simulink model "slexHARiOSExample"  (R2021a)
settings: Solver=FixedStepDiscrete  StartTime=0.0  StopTime=Inf  RelTol=1e-3
model workspace (MAT data in the model file):
  jumpingImg = [255 255 255 255 255 255 255 255 255 255 255 255 ... (960000 elements, 800x400x3)]
  runningImg = [255 255 255 255 255 255 255 255 255 255 255 255 ... (960000 elements, 800x400x3)]
  sittingImg = [255 255 255 255 255 255 255 255 255 255 255 255 ... (960000 elements, 800x400x3)]
  standingImg = [255 255 255 255 255 255 255 255 255 255 255 255 ... (960000 elements, 800x400x3)]
  walkingImg = [255 255 255 255 255 255 255 255 255 255 255 255 ... (960000 elements, 800x400x3)]
values from neighbouring files (symbols this model uses):
  X = meas(:,1:2)    [ClusteringUsingGaussianMixtureModelsExample.m]    (also in ComputePairwiseDistance2UsingACustomDistanceFunctionExample.m = rand(3,3); EstimatePosteriorClassProbabilitiesECOCExample.m = X'; FittingGaussianProcessRegressionModelsToLargeDatasetsExample.m = [X,X.^2]; ModelswithCorrelatedandUncorrelatedRandomEffectsExample.m = [ones(406,1) Acceleration Horsepower])
  Y = tsne(X,'Algorithm','barneshut','NumPCAComponents',50)    [ChangeTsneSettingsExample.m]    (also in ComputePairwiseDistance2UsingACustomDistanceFunctionExample.m = [X(:,1:2) rand(3,1)]; TSNEOutputFunctionExample.m = tsne(meas,'Options',opts,'Algorithm','exact'); TuneGaussianMixtureModelsExample.m = zeros(n,1); VisualizeHighDimensionalDataUsingTSNEExample.m)
  Z = {ones(406,1),Acceleration}    [ModelswithCorrelatedandUncorrelatedRandomEffectsExample.m]
undefined symbols (not defined in the file or in its folder): Data_Display, HAR_app_ios
libraries: iosuilib x4, iosaudiovideolib x1, iossensorlib x1
(part 1 of 2)
settings Model: Creator=The MathWorks, Inc.  LastModifiedBy=The MathWorks, Inc.
settings SolverCC: AlgebraicLoopSolver=TrustRegion  MinimalZcImpactIntegration=on
settings DataIOCC: ReturnWorkspaceOutputs=off
settings OptimizationCC: PassReuseOutputArgsAs=Individual arguments  MaxStackSize=64  EfficientTunableParamExpr=on
settings DebuggingCC: ParameterTunabilityLossMsg=error  SFMachineParentedDataDiag=warning  ArithmeticOperatorsInVariantConditions=warning
settings HardwareCC: ProdBitPerPointer=32  ProdBitPerSizeT=32  ProdBitPerPtrDiffT=32  ProdLargestAtomicInteger=Long  ProdLargestAtomicFloat=Double  ProdWordSize=32  ProdHWDeviceType=ARM Compatible->ARM Cortex
settings SFSimCC: SimUseLocalCustomCode=off  MATLABDynamicMemAlloc=off
settings RTWCC: SystemTargetFile=ert.tlc  HardwareBoard=Apple iOS Device  TLCOptions="-aInlineSetEventsForThisBaseRateFcn=TLC_FALSE -aSuppressMultiTaskScheduler=TLC_FALSE  -aRateBasedStepFcn=0"  TemplateMakefile=ert_default_tmf  GenerateReport=on  RTWUseLocalCustomCode=off  Toolchain=Xcode iOS Project  BuildConfiguration=Faster Runs  LaunchReport=on
settings CodeAppCC: ForceParamTrailComments=on  IgnoreCustomStorageClasses=off  OperatorAnnotations=on  SimulinkDataObjDesc=on  SFDataObjDesc=on  MATLABFcnDesc=on  InsertBlockDesc=on  StateflowObjectComments=on  MATLABSourceComments=on
settings ERTTargetCC: SupportVariableSizeSignals=on  RootIOFormat=Structure reference

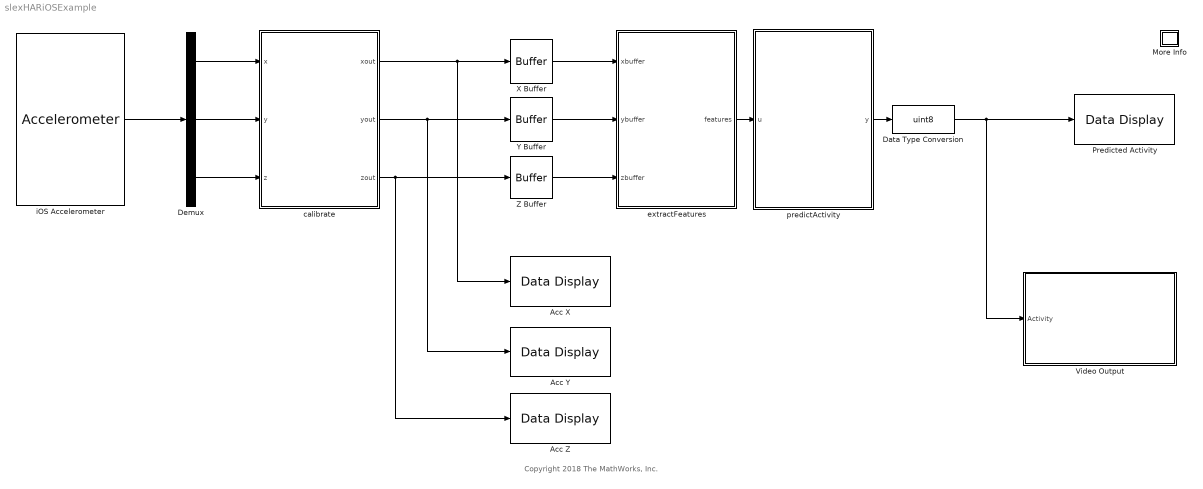
== system slexHARiOSExample ==
  note: Copyright 2018 The MathWorks, Inc.
  Acc X : iosuilib/Data Display  DataDisplayId=HAR_app_ios/X  Format=Float  Precision=6  SimulateUsing=Code generation  BlockPlatform=iOS
      settings: SourceProductBaseCode=SL_IOS
  Acc Y : iosuilib/Data Display  DataDisplayId=HAR_app_ios/Y  Format=Float  Precision=6  SimulateUsing=Code generation  BlockPlatform=iOS
      settings: SourceProductBaseCode=SL_IOS
  Acc Z : iosuilib/Data Display  DataDisplayId=HAR_app_ios/Z  Format=Float  Precision=6  SimulateUsing=Code generation  BlockPlatform=iOS
      settings: SourceProductBaseCode=SL_IOS
  Data Type Conversion : DataTypeConversion  OutDataTypeStr=uint8
  Demux : Demux  Outputs=3
  More Info : Subsystem
      settings: OpenFcn=showExample('stats/HARDeploymentExample')
      mask Display: disp('?')
  Predicted Activity : iosuilib/Data Display  DataDisplayId=HAR_app_ios/Data_Display  Format=Float  Precision=6  SimulateUsing=Code generation  BlockPlatform=iOS
      settings: SourceProductBaseCode=SL_IOS
  Video Output : Subsystem
  X Buffer : Buffer  N=32  V=12  OutputFrames=off
  Y Buffer : Buffer  N=32  V=12  OutputFrames=off
  Z Buffer : Buffer  N=32  V=12  OutputFrames=off
  calibrate : MATLAB Function  TreatAsAtomicUnit=on
  extractFeatures : MATLAB Function  TreatAsAtomicUnit=on
  iOS Accelerometer : iossensorlib/Accelerometer  OutputVector_=on  SampleTime_=0.1  blockPlatform=iOS
      settings: SourceProductBaseCode=SL_IOS
  predictActivity : MATLAB Function  TreatAsAtomicUnit=on
  wires:
  Data Type Conversion/1 -> Predicted Activity/1, Video Output/1(Activity)
  calibrate/3(zout) -> Acc Z/1, Z Buffer/1
  Y Buffer/1 -> extractFeatures/2(ybuffer)
  extractFeatures/1(features) -> predictActivity/1(u)
  X Buffer/1 -> extractFeatures/1(xbuffer)
  calibrate/2(yout) -> Acc Y/1, Y Buffer/1
  predictActivity/1(y) -> Data Type Conversion/1
  Z Buffer/1 -> extractFeatures/3(zbuffer)
  calibrate/1(xout) -> Acc X/1, X Buffer/1
  Demux/1 -> calibrate/1(x)
  Demux/3 -> calibrate/3(z)
  iOS Accelerometer/1 -> Demux/1
  Demux/2 -> calibrate/2(y)
